simulink model "Final_Railgun_discharging_model"  (R2019b)
settings: Solver=VariableStepAuto  StartTime=0.0  StopTime=10.0  RelTol=1e-3
settings Model: Creator=keato  LastModifiedBy=keato

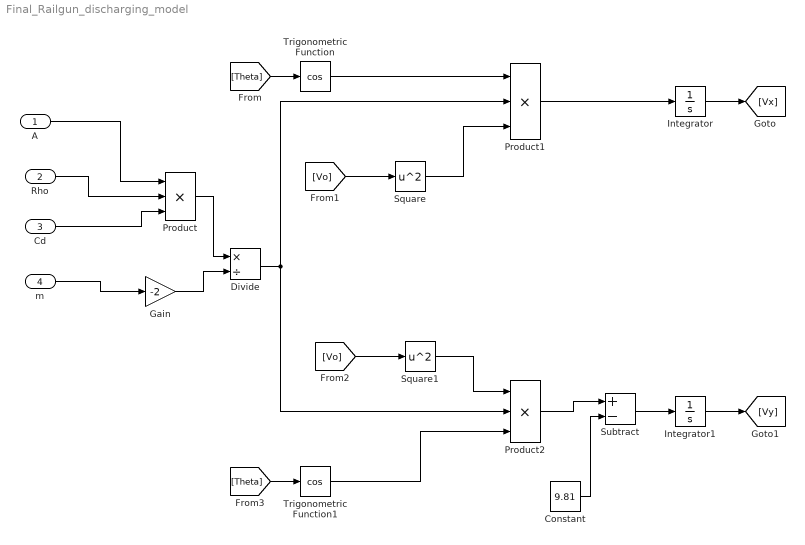
== system Final_Railgun_discharging_model ==
  A : Inport
  Rho : Inport  Port=2
  Cd : Inport  Port=3
  m : Inport  Port=4
  Constant : Constant  Value=9.81
  Divide : Product  Inputs=*/
  Gain : Gain  Gain=-2
  Integrator : Integrator
  Integrator1 : Integrator
  Product : Product  Inputs=3
  Product1 : Product  Inputs=3
  Product2 : Product  Inputs=3
  Square : Math  Operator=square  SignedPower=off  SaturateOnIntegerOverflow=on
  Square1 : Math  Operator=square  SignedPower=off  SaturateOnIntegerOverflow=on
  Subtract : Sum  Inputs=+-
  Trigonometric Function : Trigonometry  Operator=cos
  Trigonometric Function1 : Trigonometry  Operator=cos
  wires:
  A/1 -> Product/1
  Cd/1 -> Product/3
  Rho/1 -> Product/2
  Product/1 -> Divide/1
  Gain/1 -> Divide/2
  m/1 -> Gain/1
  Divide/1 -> Product2/2, Product1/2
  [Theta] -> Trigonometric Function/1
  Trigonometric Function/1 -> Product1/1
  [Vo] -> Square/1
  Square/1 -> Product1/3
  Integrator/1 -> [Vx]
  Product1/1 -> Integrator/1
  [Vo] -> Square1/1
  Square1/1 -> Product2/1
  Trigonometric Function1/1 -> Product2/3
  [Theta] -> Trigonometric Function1/1
  Product2/1 -> Subtract/1
  Constant/1 -> Subtract/2
  Subtract/1 -> Integrator1/1
  Integrator1/1 -> [Vy]
